simulink model "DCmotor"  (R2016a)
settings: Solver=ode23t  StartTime=0.0  StopTime=10.0  RelTol=1e-3  AbsTol=1e-3
model workspace (MAT data in the model file):
  rs = Simulink.Signal
  rs.DataType = 'double'
  rs.Dimensions = 1
  rs.DimensionsMode = 'Fixed'
  rs.Complexity = 'real'
  rs.SampleTime = -1
  rs.SamplingMode = 'auto'
  rs.InitialValue = '5'
libraries: fl_lib x12, nesl_utility x3
settings Model: Creator=STF2972  LastModifiedBy=STF2972
settings GRTTargetCC: GeneratePreprocessorConditionals=Use local settings
settings SimscapeCC: SimscapeLogType=all  SimscapeLogDataHistory=10000

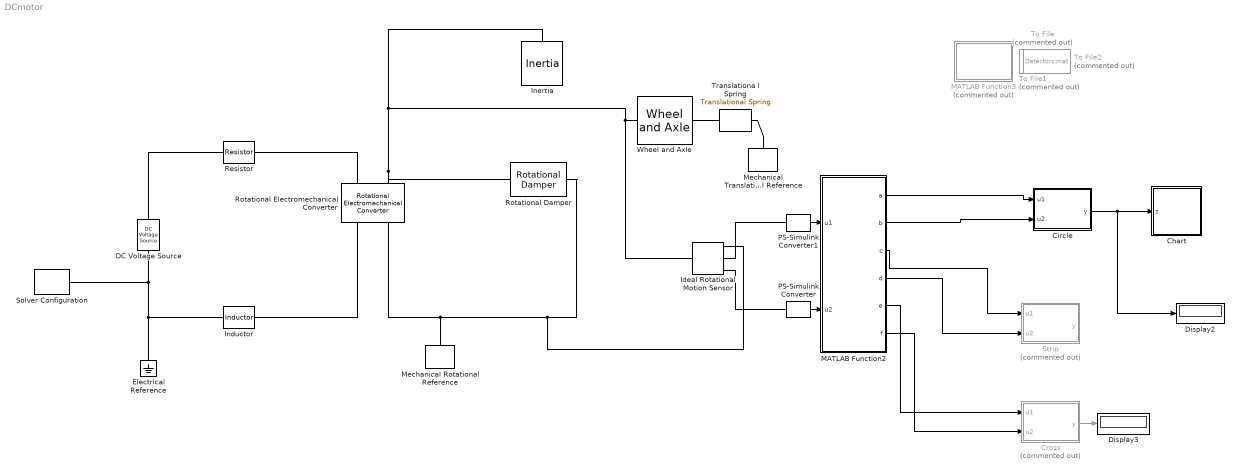
== system DCmotor ==
  Chart : Stateflow chart  TreatAsAtomicUnit=on
  Circle : MATLAB Function  TreatAsAtomicUnit=on
  Cross : MATLAB Function  Commented=on  TreatAsAtomicUnit=on
  DC Voltage Source : fl_lib/Electrical/Electrical Sources/DC Voltage Source  v0=5 V
  Display2 : Display
  Display3 : Display
  Electrical Reference : fl_lib/Electrical/Electrical Elements/Electrical Reference
  Ideal Rotational Motion Sensor : fl_lib/Mechanical/Mechanical Sensors/Ideal Rotational Motion Sensor  offset=0 rad
  Inductor : fl_lib/Electrical/Electrical Elements/Inductor  l=1e-6 H  r=0 Ohm  g=1e-9 1/Ohm  i_specify=off  i_priority=None  i=0 A  v_specify=off  v_priority=None  v=0 V  i_L_specify=off  i_L_priority=High  i_L=0 A
  Inertia : fl_lib/Mechanical/Rotational Elements/Inertia  inertia=0.2 kg*m^2  w_specify=off  w_priority=High  w=0 rad/s  t_specify=off  t_priority=None  t=0 N*m
  MATLAB Function2 : MATLAB Function  TreatAsAtomicUnit=on
  MATLAB Function3 : MATLAB Function  Commented=on  TreatAsAtomicUnit=on
  Mechanical Rotational Reference : fl_lib/Mechanical/Rotational Elements/Mechanical Rotational Reference
  Mechanical Translational Reference : fl_lib/Mechanical/Translational Elements/Mechanical Translational Reference
  PS-Simulink Converter : nesl_utility/PS-Simulink Converter  PhysicalDomain=network_engine_domain  SubClassName=ps_output  LeftPortType=input  RightPortType=output  PseudoPeriodic=off  Frequencies=[]  Unit=deg  AffineConversion=off
  PS-Simulink Converter1 : nesl_utility/PS-Simulink Converter  PhysicalDomain=network_engine_domain  SubClassName=ps_output  LeftPortType=input  RightPortType=output  PseudoPeriodic=off  Frequencies=[]  Unit=1  AffineConversion=off
  Resistor : fl_lib/Electrical/Electrical Elements/Resistor  R=.1 Ohm  i_specify=off  i_priority=None  i=0 A  v_specify=off  v_priority=None  v=0 V
  Rotational Electromechanical Converter : fl_lib/Electrical/Electrical Elements/Rotational Electromechanical Converter  K=0.1 V/(rad/s)  i_specify=off  i_priority=None  i=0 A  v_specify=off  v_priority=None  v=0 V  t_specify=off  t_priority=None  t=0 N*m  w_specify=off  w_priority=None  w=0 rad/s
  Rotational Damper : fl_lib/Mechanical/Rotational Elements/Rotational Damper  D=0.2 N*m/(rad/s)  w_specify=off  w_priority=None  w=0 rad/s  t_specify=off  t_priority=None  t=0 N*m
  Solver Configuration : nesl_utility/Solver Configuration  PhysicalDomain=network_engine_domain  SubClassName=solver  LeftPortType=input  RightPortType=generic  Accelerate=off  Tones=[]  Harmonics=[]  SimulateNoise=off  Profile=off  UseLocalSampling=off  EnableSwitchedLinearOptims=on  FrequencyDomain=off  UseCCode=off  RelTol=0.001  AbsTol=1e-06  MinStep=1e-09  ToWorkspace=off  RevertToSquareIcSolve=off  NumHomotopyIterations=100  PhasorMode=off  PhasorModeNumHarmonics=1  OverrideAbsTol=off  DoDC=off  ResidualTolerance=1e-09  UseLocalSolver=off  LocalSolverChoice=NE_BACKWARD_EULER_ADVANCER  LocalSolverSampleTime=0.001  DoFixedCost=off  MaxNonlinIter=3  MaxModeIter=2  LinearAlgebra=Sparse  DelaysMemoryBudget=1024  AutomaticFiltering=on  FilteringTimeConstant=0.001
  Strip : MATLAB Function  Commented=on  TreatAsAtomicUnit=on
  To File : ToFile  Commented=on  Filename=u1.mat  MatrixName=u_1
  To File1 : ToFile  Commented=on  Filename=u2.mat  MatrixName=u_2
  To File2 : ToFile  Commented=on  Filename=Detectors.mat  MatrixName=detectorSet
  Translationa l Spring : fl_lib/Mechanical/Translational Elements/Translational Spring  spr_rate=1000 N/m  v_specify=off  v_priority=None  v=0 m/s  f_specify=off  f_priority=None  f=0 N  x_specify=off  x_priority=High  x=0 m
  Wheel and Axle : fl_lib/Mechanical/Mechanisms/Wheel and Axle  R=0.03 m  or=1  t_specify=off  t_priority=None  t=0 N*m  f_specify=off  f_priority=None  f=0 N
  wires:
  PS-Simulink Converter/1 -> MATLAB Function2/2(u2)
  PS-Simulink Converter1/1 -> MATLAB Function2/1(u1)
  MATLAB Function2/2(b) -> Circle/2(u2)
  MATLAB Function2/1(a) -> Circle/1(u1)
  MATLAB Function2/3(c) -> Strip/1(u1)
  MATLAB Function2/4(d) -> Strip/2(u2)
  MATLAB Function2/5(e) -> Cross/1(u1)
  MATLAB Function2/6(f) -> Cross/2(u2)
  Circle/1(y) -> Display2/1, Chart/1(z)
  Cross/1(y) -> Display3/1
  connections:
  DC Voltage Source/LConn1 -- Resistor/LConn1
  Resistor/RConn1 -- Rotational Electromechanical Converter/LConn1
  DC Voltage Source/RConn1 -- Solver Configuration/RConn1 -- Electrical Reference/LConn1 -- Inductor/LConn1
  Inductor/RConn1 -- Rotational Electromechanical Converter/RConn1
  Rotational Electromechanical Converter/RConn2 -- Ideal Rotational Motion Sensor/RConn1 -- Rotational Damper/RConn1 -- Mechanical Rotational Reference/LConn1
  Rotational Electromechanical Converter/LConn2 -- Ideal Rotational Motion Sensor/LConn1 -- Wheel and Axle/LConn1 -- Inertia/LConn1 -- Rotational Damper/LConn1
  Translationa l Spring/LConn1 -- Wheel and Axle/RConn1
  Mechanical Translational Reference/LConn1 -- Translationa l Spring/RConn1
  Ideal Rotational Motion Sensor/RConn3 -- PS-Simulink Converter/LConn1
  Ideal Rotational Motion Sensor/RConn2 -- PS-Simulink Converter1/LConn1

== matlab function DCmotor/Circle ==
  data: u1 input; u2 input; y output [0..50]; rs data_store_memory
function y = fcn(u1, u2)
%% #codegen
coder.extrinsic('UseKnnSearch');
persistent detSet p Y N  x n z z_alpha training testing;

coder.varsize('detSet',[30000000 3]);
coder.varsize('Y',[30000000 2]);
coder.varsize('X',[30000000 2]);
%
if isempty(N)&&isempty(x)&&isempty(n)
N=0; % count of not self
detSet=[0 0 0] 
Y=[u1 u2];
x=0; % count of not self 
p=0.9; % default probability 
n =(max(5/p, 5/(1-p)));
 % sample size/ total number of data
% detected occurances
z_alpha =3.49;
z=0;
testing =false;
training =false;
end

if size(Y,1)<200
    Y =[Y; [u1 u2]];
%  Y=[Y; [round(u1*1000)/1000 round(u2*1000)/1000]];
%  Y =unique(Y,'rows');
 
else
 training =true; 

end 

if (training)
    
 if z<z_alpha
    % Randomly generate a,b
    r = randi([0 100],1,2);
    a=r(1);
    b=r(2);
    d=0;
    e=0;
    %find the closest self point 
    [e,d]=UseKnnSearch(Y,[a,b]);
 if d>1
       N =N+1;  
    if (size(detSet,1) >2)
         %find the closest detector
           X = detSet(: , 1:2) ;
           ee=0;
           dd=0;
          [ee,dd]=UseKnnSearch(X,[a,b]);          
          if (dd> detSet(ee, 3))&& ~(N==n)
              %covered =false; 
              detSet=[detSet; [a b d]];
              circle(a,b,d); 
%               x =x+1;
          else
              if (N==n)
                  %%  why nonself point x is set to zero
                  %A hypothesis test is a statistical test that is used to determine 
                  %whether there is enough evidence in a sample of data to infer
                  %that a certain condition is true for the entire population.
                 N=0;
                 x=0;
              else
              %covered =true;
                x=x+1;
               % p =x/n; % probability of not self
                q= 1-p;
                z=x/sqrt(n*p*q)-sqrt(n*p/q);
                % evaluate z score
                if ~(z<z_alpha)
                    testing =true;
                end
                    
              end      
          end            
    else
        %first detector
       detSet=[detSet; [a b d]]; 
       circle(a,b,d); 
    end
 
 end 
 end 
end 

if(testing)  
    X = detSet(: , 1:2) ;
    [ee,dd]=UseKnnSearch(X,[u1,u2]);
    %ee index of X which has the value of the nearest and dd is the
    %distance between the two points
          if (dd< detSet(ee,3))  
               plot(u1 ,u2 , '.r', 'MarkerSize',09);
              drawnow;
              
          end 
end 
 testing  
y =z;
 
 
function circle(x,y,r)
%x and y are the coordinates of the center of the circle
%r is the radius of the circle
%0.01 is the angle step, bigger values will draw the circle faster but
%you might notice imperfections (not very smooth)
ang=0:0.01:2*pi; 
xp=r*cos(ang);
yp=r*sin(ang);
plot(x+xp,y+yp);
drawnow;
hold on

== stateflow chart DCmotor/Chart ==
  state Testing
    state Transient
    (default) -> Transient
  state Training
    state Steady
    (default) -> Steady
  (default) -> Training
  Training -> Testing : [z>3.49]
  data: z input

== matlab function DCmotor/MATLAB Function2 ==
  data: u1 input; a output; u2 input; b output; c output; d output; e output; f output
function [a,b,c, d,e,f] = createSelf(u1,u2)
%#codegen
% global rs ;
%Boundary aware V-detector system

% str = {'circle', 'cross', 'triangle','ring', 'stripe', 'intersection', 'pentagram'} ;
% s = (listdlg('PromptString','Select a file:',...
%                 'SelectionMode','single',...
%                 'ListString',str));

% if s ==circle
    
% end 
%% Circle


%% Cross
% Thickness and location of the cross
% if the point is between x1, x2 and y1,y2 ; the point is discarded 
plot(u1,u2);
%% Triangle
% Size (radius of circumscribed circle)
% points 
%% Ring 
% Out and inner radius
% two radii
%% Stripe 
% Width
% x1, x2 or y1, y2
%% Intersection 
% cross size and location , circle radius
% radius and cross
%% Pentagram 
% side (radius of circumscribed circle)

a = u1;
b=u2 ;
c=u1;
d=u2;
e=u1;
f=u2;

== matlab function DCmotor/MATLAB Function3 ==
  data: rs data_store_memory; x1 data_store_memory; x2 data_store_memory; y1 data_store_memory; y2 data_store_memory
function setGlobals
%#codegen
global rs;
rs =5;


    function r =getRs
        global rs;
        r=rs;

== matlab function DCmotor/Strip ==
  data: u1 input; y output; u2 input
function y = Strip(u1,u2)

%% #codegen
coder.extrinsic('clc');
persistent detSet N  m n x1 x2;
coder.varsize('detSet',[30000000 3]);   
if isempty(N)
    
x2=5;
  x1=-5;

        if (u1<x1)
            toself =abs(x1-u1);
        else
            toself =abs(x2-u1);
        end 
        detSet=[u1 u2 toself];
         circle(u1,u2,toself);
   
%%Distance measures
end
 
if isempty(N)&&isempty(m)&&isempty(n)
N=0; % count of not self

m=0; % count of not self 
p=0.5; % default probability 
n =(max(5/p, 5/(1-p)));
 % sample size/ total number of data
% detected occurances

end

z_alpha =3.49;
 
% Estimated coverage 99% 
%%%% Hyppthesis testing %%%%

% Sample a point 



% %%
% %two dimensional space 
 
 a=u1;
 b =u2;
 


 if(a>0.1 && b>0.1) % to reduce the noise ???     
    if (N<n) % exit criterion 
        n =n+1; % count the sample size
        if~(a>x1 && a<x2) %  -non self
        %%--------not-self-------
        %% 
       
        
        if (a<x1)
            toself =abs(x1-a);
        else
            toself =abs(x2-a);
        end 
        
        N=N+1; % count (non-self) sample
         
%         if size(detSet,1)==1 % first detector    
%             % addthe first detector to the map
%             c=sqrt(((b-c_s2)^2+(a-c_s1)^2))-rs;
%             detSet=[detSet; [a b c]];
%             %y=detSet;
%             %xlswrite('detectors.xlsx',detSet);
%            
%             circle(a,b,c);                 
%         else
        %find the closest detector
        rDet=0;       
          covered=false;
           dist_min = (b-detSet(1,2))^2+(a-detSet(1,1))^2;
          if size(detSet,1) >2
             % The point is covered by an existing detector 
            %finding the minimum distance to the point selected
             % distance from self
            for j=2: size(detSet,1)                                             
                    temp_dist=(b-detSet(j,2))^2+(a-detSet(j,1))^2;
                    if (abs (sqrt(((b-detSet(j,2))^2+(a-detSet(j,1))^2))-detSet(j,3))>detSet(j,3)) 
                        if(temp_dist<dist_min)
                        dist_min=temp_dist;
                        rDet =detSet(j,3);
                        end 
                    else
                        covered =true;
                    end
                    
            end 
                %% check if it is out side of the closest detector                             
            %Check if it is within the raduis of the closest detector
          end    
        
            %% Covered? yes 
            if (rDet>dist_min && rDet>0) || covered
                 %% Covered? yes
                m=m+1; % count covered sample
                p =N/n; % probability of not self
                q= 1-p;
                z=m/sqrt(n*p*q)-sqrt(n*p/q); % evaluate z score
                if z<z_alpha % not enough coverage
                    if(N==n) 
                        %% Accept all saved candidates as new detectors
                        N=0;
                        m=0;
                    
                        
                    end 
                else %enough coverage
                    N=n+1; % exist the function
                end 
            else 
                %% Covered? No : save the candidate
               
                    detSet=[detSet; [a b toself]];
                    circle(a,b,toself);
                
               
              
                   
               
           % end    
            end 
        detSet
        end 
       
    end 
 
 end 

y =u1;

function circle(x,y,r)
%x and y are the coordinates of the center of the circle
%r is the radius of the circle
%0.01 is the angle step, bigger values will draw the circle faster but
%you might notice imperfections (not very smooth)
ang=0:0.01:2*pi; 
xp=r*cos(ang);
yp=r*sin(ang);
plot(x+xp,y+yp);
hold on;

function h = filledCircle(center,r,N,color)
THETA=linspace(0,2*pi,N);
RHO=ones(1,N)*r;
[X,Y] = pol2cart(THETA,RHO);
X=X+center(1);
Y=Y+center(2);
h=fill(X,Y,color);
axis square;

== matlab function DCmotor/Cross ==
  data: u1 input; y output; u2 input
function y = Cross(u1,u2)
%% #codegen
coder.extrinsic('clc');
persistent detSet N  m n x1 x2 y1 y2;
if isempty(N)
    
y1=31.83098862;
y2 =32.83098862;


x2=1;
x1=-1; 
%%Distance measures

 
end
coder.varsize('detSet',[30000000 3]);
% dist_min=0;
% temp_dist=0;
% rDet=0;
%drawCircle(c_s1, c_s2,rs);
%filledCircle([c_s1,c_s2],rs,1000,'r')
%Until N ==m_max
if isempty(N)&&isempty(m)&&isempty(n)
N=0; % count of not self
 
m=0; % count of not self 
p=0.5; % default probability 
n =(max(5/p, 5/(1-p)));
 % sample size/ total number of data
% detected occurances

end

z_alpha =3.49;
 
% Estimated coverage 99% 
%%%% Hyppthesis testing %%%%

% Sample a point 



% %%
% %two dimensional space 
 
 a=u1;
 b =u2;
 


 if(a>0.1 && b>0.1) % to reduce the noise ???     
    if (N<n) % exit criterion 
        n =n+1; % count the sample size
        if~(a>x1 && a<x2 &&b>y1 && b<y2 )  %  -non self
        %%--------not-self-------
        %% 
        if (a<x1)
            if (b>y2)
            if abs(b-y2)<abs(a-x1)
            toself =abs(x1-a);
            else
             toself =abs(y2-b);
            end 
            else
               if abs(b-y2)<abs(a-x1)
                toself =abs(x1-a);
               else
                toself =abs(y2-b);
            end 
            end
            
        else
            toself =abs(x2-a);
        end 
        toself =sqrt(((b-c_s2)^2+(a-c_s1)^2))-rs;
        detSet= [
        N=N+1; % count (non-self) sample
         
%         if size(detSet,1)==1 % first detector    
%             % addthe first detector to the map
%             c=sqrt(((b-c_s2)^2+(a-c_s1)^2))-rs;
%             detSet=[detSet; [a b c]];
%             %y=detSet;
%             %xlswrite('detectors.xlsx',detSet);
%            
%             circle(a,b,c);                 
%         else
        %find the closest detector
           rDet=0;       
           covered=false; % The point is covered by an existing detector 
            %finding the minimum distance to the point selected
             dist_min = (b-detSet(1,2))^2+(a-detSet(1,1))^2; % distance from self
            for j=2: size(detSet,1)                                             
                    temp_dist=(b-detSet(j,2))^2+(a-detSet(j,1))^2;
                    if (abs (sqrt(((b-detSet(j,2))^2+(a-detSet(j,1))^2))-detSet(j,3))>detSet(j,3)) 
                        if(temp_dist<dist_min)
                        dist_min=temp_dist;
                        rDet =detSet(j,3);
                        end 
                    else
                        covered =true;
                    end
                    
            end 
                %% check if it is out side of the closest detector                             
            %Check if it is within the raduis of the closest detector
            
        
            %% Covered? yes 
            if rDet>sqrt(dist_min) || covered
                 %% Covered? yes
                m=m+1; % count covered sample
                p =N/n; % probability of not self
                q= 1-p;
                z=m/sqrt(n*p*q)-sqrt(n*p/q); % evaluate z score
                if z<z_alpha % not enough coverage
                    if(N==n) 
                        %% Accept all saved candidates as new detectors
                        N=0;
                        m=0;                       
                    end 
                else %enough coverage
                    N=n+1; % exist the function
                end 
            else 
                %% Covered? No : save the candidate
               
                if toself < sqrt(dist_min)
                    detSet=[detSet; [a b toself]];
                    circle(a,b,toself);
                else
                    detSet=[detSet; [a b sqrt(dist_min)]];
                    circle(a,b,sqrt(dist_min));
                end
               
                detSet
               
           % end    
        end 
        end 
       
    end 
 end 

y =a;
 
 

 function circle(x,y,r)
%x and y are the coordinates of the center of the circle
%r is the radius of the circle
%0.01 is the angle step, bigger values will draw the circle faster but
%you might notice imperfections (not very smooth)
ang=0:0.01:2*pi; 
xp=r*cos(ang);
yp=r*sin(ang);
plot(x+xp,y+yp);
hold on

function h = filledCircle(center,r,N,color)
THETA=linspace(0,2*pi,N);
RHO=ones(1,N)*r;
[X,Y] = pol2cart(THETA,RHO);
X=X+center(1);
Y=Y+center(2);
h=fill(X,Y,color);
axis square;
